simulink model "mrefrobotarm_modified_previous_y_previous_u_previous_ref"  (R2018b)
settings: Solver=FixedStepAuto  StartTime=0.0  StopTime=10  RelTol=1e-3  AbsTol=1e-6
undefined symbols (not defined in the file or in its folder): options, sfunxy2
libraries: neural x949, simulink x1
(part 25 of 31)

== system mrefrobotarm_modified_previous_y_previous_u_previous_ref/good_one/Layer 2/LW{2,1} ==
  "ad{2,1}" : Inport  PortDimensions=40
      mask Display: e = 0.06;c1 = [120 230 180]/255;c2 = ([120 230 180]+0)/(256+128);c3 = ([120 230 180]+128)/(256+128);patch([0 1 1 0],[0 0 1 1],c1);patch([0 1 1 1-e 1-e 0+e],[0 0 1 1-e 0+e 0+e],c2);patch([0 0 1 1-e 0+e 0+e],[0 1 1 1-e 1-e 0+e],c3);plot([0 1 1 0 0],[0 0 1 1 0]);
  "IW{2,1}(1,:)'" : Constant  Value=[-0.016177229018260623483183024973186547867953777313232421875;-0.096537565963239924116123802377842366695404052734375;-0.057321807043975082918141339405337930656969547271728515625;-0.33528888680619395312731967351282946765422821044921875;0.254536930512510084501087703756638802587985992431640625;0.160443440271881343495152805189718492329120635986328125;0.0298865770847444554847438524802782922051846981048583984375;-0.4905367415926971119688460021279752254486083984375;0.26949914824714371608394003487774170935153961181640625;0.279888712410184592460637986732763238251209259033203125;0.156475783700833093181614685818203724920749664306640625;0.427246473409241656060686409546178765594959259033203125;0.24892939455984686158984686699113808572292327880859375;0.2130922585627052778800560872696223668754100799560546875;0.09388320364746434443237177447372232563793659210205078125;-0.159198518445238190732737848520628176629543304443359375;0.01438968371043083081806113199263563728891313076019287109375;-0.0623226293562786637370010112135787494480609893798828125;0.403201394446350114275645637462730519473552703857421875;-1.209114934242264904895591826061718165874481201171875;0.8556447732028324981712330554728396236896514892578125;-0.124638437957925785060098178291809745132923126220703125;-0.87136147182802703436976798911928199231624603271484375;0.68733337340105526980238437317893840372562408447265625;0.08171188805447136827009302351143560372292995452880859375;0.62154317245998480512270134568098001182079315185546875;-0.142201082792390798292814224623725749552249908447265625;-0.058134677163346359929363416085834614932537078857421875;-0.0164424917618185388590301698741313884966075420379638671875;0.0377358747014499840144452491585980169475078582763671875;0.292289912994841805105039611589745618402957916259765625;0.76420559375889940412207579356618225574493408203125;-0.03434516763233952385547809171839617192745208740234375;-0.037602080927664947862520961052723578177392482757568359375;0.006550485557210122648796879474275556276552379131317138671875;0.04940602468184761286718043038490577600896358489990234375;-0.1541501906398750343374359772496973164379596710205078125;0.01187461167243125149950433439016705960966646671295166015625;0.01447827447317109363089659979095813469029963016510009765625;0.0172233274061301920576649848726447089575231075286865234375]
      mask Display: e = 0.06;c1 = [120 150 230]/255;c2 = ([120 150 230]+0)/383;c3 = ([120 150 230]+128)/383;patch([0 1 1 0],[0 0 1 1],c1);patch([0 1 1 1-e 1-e 0+e],[0 0 1 1-e 0+e 0+e],c2);patch([0 0 1 1-e 0+e 0+e],[0 1 1 1-e 1-e 0+e],c3);plot([0 1 1 0 0],[0 0 1 1 0]);disp('weights');
  Mux : Mux  Inputs=1
      mask Display: e = 0.06;c1 = [120 150 230]/255;c2 = ([120 150 230]+0)/383;c3 = ([120 150 230]+128)/383;patch([0 1 1 0],[0 0 1 1],c1);patch([0 1 1 1-e 1-e 0+e],[0 0 1 1-e 0+e 0+e],c2);patch([0 0 1 1-e 0+e 0+e],[0 1 1 1-e 1-e 0+e],c3);plot([0 1 1 0 0],[0 0 1 1 0]);disp('Mux');
  dotprod1 : neural/Weight Functions/dotprod
  "lz{2,1}" : Outport
      mask Display: e = 0.06;c1 = [120 230 180]/255;c2 = ([120 230 180]+0)/(256+128);c3 = ([120 230 180]+128)/(256+128);patch([0 1 1 0],[0 0 1 1],c1);patch([0 1 1 1-e 1-e 0+e],[0 0 1 1-e 0+e 0+e],c2);patch([0 0 1 1-e 0+e 0+e],[0 1 1 1-e 1-e 0+e],c3);plot([0 1 1 0 0],[0 0 1 1 0]);
  wires:
  "IW{2,1}(1,:)'"/1 -> dotprod1/1
  "ad{2,1}"/1 -> dotprod1/2
  dotprod1/1 -> Mux/1
  Mux/1 -> "lz{2,1}"/1

== system mrefrobotarm_modified_previous_y_previous_u_previous_ref/no_ss_error/Layer 1/Delays 1 ==
  "p{1}" : Inport  PortDimensions=10
      mask Display: e = 0.06;c1 = [120 230 180]/255;c2 = ([120 230 180]+0)/(256+128);c3 = ([120 230 180]+128)/(256+128);patch([0 1 1 0],[0 0 1 1],c1);patch([0 1 1 1-e 1-e 0+e],[0 0 1 1-e 0+e 0+e],c2);patch([0 0 1 1-e 0+e 0+e],[0 1 1 1-e 1-e 0+e],c3);plot([0 1 1 0 0],[0 0 1 1 0]);
  mux : Mux  Inputs=1
      mask Display: e = 0.06;c1 = [120 150 230]/255;c2 = ([120 150 230]+0)/383;c3 = ([120 150 230]+128)/383;patch([0 1 1 0],[0 0 1 1],c1);patch([0 1 1 1-e 1-e 0+e],[0 0 1 1-e 0+e 0+e],c2);patch([0 0 1 1-e 0+e 0+e],[0 1 1 1-e 1-e 0+e],c3);plot([0 1 1 0 0],[0 0 1 1 0]);disp('Mux')
  "pd{1,1}" : Outport
      mask Display: e = 0.06;c1 = [120 230 180]/255;c2 = ([120 230 180]+0)/(256+128);c3 = ([120 230 180]+128)/(256+128);patch([0 1 1 0],[0 0 1 1],c1);patch([0 1 1 1-e 1-e 0+e],[0 0 1 1-e 0+e 0+e],c2);patch([0 0 1 1-e 0+e 0+e],[0 1 1 1-e 1-e 0+e],c3);plot([0 1 1 0 0],[0 0 1 1 0]);
  wires:
  "p{1}"/1 -> mux/1
  mux/1 -> "pd{1,1}"/1

== system mrefrobotarm_modified_previous_y_previous_u_previous_ref/no_ss_error/Layer 1/IW{1,1} ==
  "pd{1,1}" : Inport  PortDimensions=10
      mask Display: e = 0.06;c1 = [120 230 180]/255;c2 = ([120 230 180]+0)/(256+128);c3 = ([120 230 180]+128)/(256+128);patch([0 1 1 0],[0 0 1 1],c1);patch([0 1 1 1-e 1-e 0+e],[0 0 1 1-e 0+e 0+e],c2);patch([0 0 1 1-e 0+e 0+e],[0 1 1 1-e 1-e 0+e],c3);plot([0 1 1 0 0],[0 0 1 1 0]);
  "IW{1,1}(1,:)'" : Constant  Value=[0.52268284589696356601251636675442568957805633544921875;0.26452162295619441323424325673840939998626708984375;0.6302383946003129455704083738964982330799102783203125;0.1670856108177140864068377368312212638556957244873046875;1.6390040056115242617096328103798441588878631591796875;-0.8986878651207874657558249964495189487934112548828125;-1.114512508252162081845426655490882694721221923828125;-0.423456516896269619110171333886682987213134765625;0.20198751257098113143229056731797754764556884765625;0.47139361413845304316083684170735068619251251220703125]
      mask Display: e = 0.06;c1 = [120 150 230]/255;c2 = ([120 150 230]+0)/383;c3 = ([120 150 230]+128)/383;patch([0 1 1 0],[0 0 1 1],c1);patch([0 1 1 1-e 1-e 0+e],[0 0 1 1-e 0+e 0+e],c2);patch([0 0 1 1-e 0+e 0+e],[0 1 1 1-e 1-e 0+e],c3);plot([0 1 1 0 0],[0 0 1 1 0]);disp('Weights');
  "IW{1,1}(10,:)'" : Constant  Value=[1.2597231626400127169063125620596110820770263671875;0.331393970410923388580926030044793151319026947021484375;-0.052791829980691880319643161101339501328766345977783203125;0.3149576319875482255383758456446230411529541015625;0.55511068393909435148003694848739542067050933837890625;0.96721718074699747358380363948526792228221893310546875;0.9771018529696899879155580492806620895862579345703125;-0.269806974086425788161847094670520164072513580322265625;1.5151280312247499271194328684941865503787994384765625;-0.1203640526482755712667227498968713916838169097900390625]
      mask Display: e = 0.06;c1 = [120 150 230]/255;c2 = ([120 150 230]+0)/383;c3 = ([120 150 230]+128)/383;patch([0 1 1 0],[0 0 1 1],c1);patch([0 1 1 1-e 1-e 0+e],[0 0 1 1-e 0+e 0+e],c2);patch([0 0 1 1-e 0+e 0+e],[0 1 1 1-e 1-e 0+e],c3);plot([0 1 1 0 0],[0 0 1 1 0]);disp('Weights');
  "IW{1,1}(11,:)'" : Constant  Value=[-1.0743295819324780726589096957468427717685699462890625;1.1501577563757912070485645017470233142375946044921875;-0.86958362725818016958356793111306615173816680908203125;0.29387617229097073856536326275090686976909637451171875;1.8821297501686731212799941204139031469821929931640625;-0.8969617337271689194722057436592876911163330078125;-0.153795010052089897722993327988660894334316253662109375;-0.424733827549765796671721318489289842545986175537109375;1.58320681511508354333273018710315227508544921875;0.1647340537904307955496818749452359043061733245849609375]
      mask Display: e = 0.06;c1 = [120 150 230]/255;c2 = ([120 150 230]+0)/383;c3 = ([120 150 230]+128)/383;patch([0 1 1 0],[0 0 1 1],c1);patch([0 1 1 1-e 1-e 0+e],[0 0 1 1-e 0+e 0+e],c2);patch([0 0 1 1-e 0+e 0+e],[0 1 1 1-e 1-e 0+e],c3);plot([0 1 1 0 0],[0 0 1 1 0]);disp('Weights');
  "IW{1,1}(12,:)'" : Constant  Value=[-0.180456952373312662363247227403917349874973297119140625;-0.9119322220681633783812003457569517195224761962890625;-0.7206769917408870629316197664593346416950225830078125;0.51991005391813416292023930509458296000957489013671875;1.3325131012939082086887765399296768009662628173828125;1.2068826405339387886073154732002876698970794677734375;-0.25797017784359310699215939166606403887271881103515625;-0.5702990169558226352108931678230874240398406982421875;-1.0030700930944382864851149861351586878299713134765625;-0.8022722469174292658777858378016389906406402587890625]
      mask Display: e = 0.06;c1 = [120 150 230]/255;c2 = ([120 150 230]+0)/383;c3 = ([120 150 230]+128)/383;patch([0 1 1 0],[0 0 1 1],c1);patch([0 1 1 1-e 1-e 0+e],[0 0 1 1-e 0+e 0+e],c2);patch([0 0 1 1-e 0+e 0+e],[0 1 1 1-e 1-e 0+e],c3);plot([0 1 1 0 0],[0 0 1 1 0]);disp('Weights');
  "IW{1,1}(13,:)'" : Constant  Value=[1.587500865720722575957779554300941526889801025390625;-0.4136221707058511665167088722228072583675384521484375;-0.52639486621294195867193366211722604930400848388671875;0.6173652998952949833011416558292694389820098876953125;0.3804309528306466514635530984378419816493988037109375;0.43292517299477883963021440649754367768764495849609375;-0.059184167845455604162197005280177108943462371826171875;-0.520069104891264455403643296449445188045501708984375;-0.262239897051457171439636795184924267232418060302734375;0.04362502873940894698723269584661466069519519805908203125]
      mask Display: e = 0.06;c1 = [120 150 230]/255;c2 = ([120 150 230]+0)/383;c3 = ([120 150 230]+128)/383;patch([0 1 1 0],[0 0 1 1],c1);patch([0 1 1 1-e 1-e 0+e],[0 0 1 1-e 0+e 0+e],c2);patch([0 0 1 1-e 0+e 0+e],[0 1 1 1-e 1-e 0+e],c3);plot([0 1 1 0 0],[0 0 1 1 0]);disp('Weights');
  "IW{1,1}(14,:)'" : Constant  Value=[0.15678260333455951158754260177374817430973052978515625;-0.2830214288855901205721465885289944708347320556640625;-0.57337904103334758065813048233394511044025421142578125;-0.58607875125629771417834490421228110790252685546875;0.9772944325289447675686460570432245731353759765625;-1.0061880783424668184267147807986475527286529541015625;0.12184461872279016281250818565240479074418544769287109375;-0.093833824658861642031837391186854802072048187255859375;0.5364472996047109365491678545367904007434844970703125;0.324149798798010035927319449911010451614856719970703125]
      mask Display: e = 0.06;c1 = [120 150 230]/255;c2 = ([120 150 230]+0)/383;c3 = ([120 150 230]+128)/383;patch([0 1 1 0],[0 0 1 1],c1);patch([0 1 1 1-e 1-e 0+e],[0 0 1 1-e 0+e 0+e],c2);patch([0 0 1 1-e 0+e 0+e],[0 1 1 1-e 1-e 0+e],c3);plot([0 1 1 0 0],[0 0 1 1 0]);disp('Weights');
  "IW{1,1}(15,:)'" : Constant  Value=[-0.597168529912007528537287726067006587982177734375;-0.26877976344490683846544243351672776043415069580078125;-0.4210029627419034081725612850277684628963470458984375;-0.895478281549339616418592413538135588169097900390625;-0.185230952547398686203194984045694582164287567138671875;-0.202950183795940486408682090768706984817981719970703125;0.57595042618450376092908982172957621514797210693359375;-0.63455501901511734974548062382382340729236602783203125;-0.979057802580790781377118037198670208454132080078125;-0.886842867770659015747014564112760126590728759765625]
      mask Display: e = 0.06;c1 = [120 150 230]/255;c2 = ([120 150 230]+0)/383;c3 = ([120 150 230]+128)/383;patch([0 1 1 0],[0 0 1 1],c1);patch([0 1 1 1-e 1-e 0+e],[0 0 1 1-e 0+e 0+e],c2);patch([0 0 1 1-e 0+e 0+e],[0 1 1 1-e 1-e 0+e],c3);plot([0 1 1 0 0],[0 0 1 1 0]);disp('Weights');
  "IW{1,1}(16,:)'" : Constant  Value=[-1.4434083519231160064322239122702740132808685302734375;-0.89746723355772584085343623883090913295745849609375;0.468903432219882787546083591223577968776226043701171875;0.5235125480188809188319964960101060569286346435546875;1.030194455855783619568910580710507929325103759765625;0.2410749054790011225435364394797943532466888427734375;-0.020026318196021346274005026089071179740130901336669921875;0.12832652380476472497861095689586363732814788818359375;0.1470700867800898148374244556180201470851898193359375;0.9743179738880478613083369054947979748249053955078125]
      mask Display: e = 0.06;c1 = [120 150 230]/255;c2 = ([120 150 230]+0)/383;c3 = ([120 150 230]+128)/383;patch([0 1 1 0],[0 0 1 1],c1);patch([0 1 1 1-e 1-e 0+e],[0 0 1 1-e 0+e 0+e],c2);patch([0 0 1 1-e 0+e 0+e],[0 1 1 1-e 1-e 0+e],c3);plot([0 1 1 0 0],[0 0 1 1 0]);disp('Weights');
  "IW{1,1}(17,:)'" : Constant  Value=[-1.998604254806128910360030204174108803272247314453125;0.781327841746925155774761151405982673168182373046875;1.104473632181291353759888806962408125400543212890625;0.6244245059941342379516981964115984737873077392578125;-1.8270110679777420426006528941798023879528045654296875;1.57781831173188979988708524615503847599029541015625;0.17040001620197653409150007064454257488250732421875;0.343192753239213887983538597836741246283054351806640625;0.3575702811109369161357562916236929595470428466796875;-0.040126214462137231586691399343180819414556026458740234375]
      mask Display: e = 0.06;c1 = [120 150 230]/255;c2 = ([120 150 230]+0)/383;c3 = ([120 150 230]+128)/383;patch([0 1 1 0],[0 0 1 1],c1);patch([0 1 1 1-e 1-e 0+e],[0 0 1 1-e 0+e 0+e],c2);patch([0 0 1 1-e 0+e 0+e],[0 1 1 1-e 1-e 0+e],c3);plot([0 1 1 0 0],[0 0 1 1 0]);disp('Weights');
  "IW{1,1}(18,:)'" : Constant  Value=[0.86997594199966099548504416816285811364650726318359375;-0.892679254067974436992471964913420379161834716796875;-0.04449260537774453461157264655412291176617145538330078125;0.9604625897041871862569450968294404447078704833984375;-0.30233191807039239140664221849874593317508697509765625;-1.8516467076794871360334582277573645114898681640625;1.262375674633811950542394697549752891063690185546875;0.28182724484288634858586419795756228268146514892578125;-0.58009991273124372757052924498566426336765289306640625;0.23561111386226318842318505630828440189361572265625]
      mask Display: e = 0.06;c1 = [120 150 230]/255;c2 = ([120 150 230]+0)/383;c3 = ([120 150 230]+128)/383;patch([0 1 1 0],[0 0 1 1],c1);patch([0 1 1 1-e 1-e 0+e],[0 0 1 1-e 0+e 0+e],c2);patch([0 0 1 1-e 0+e 0+e],[0 1 1 1-e 1-e 0+e],c3);plot([0 1 1 0 0],[0 0 1 1 0]);disp('Weights');
  "IW{1,1}(19,:)'" : Constant  Value=[-0.32234142998081638520346814402728341519832611083984375;-0.17724685528195960326769409221014939248561859130859375;0.91705950576351480396652959825587458908557891845703125;0.51157014029427372303615584314684383571147918701171875;0.1887748557125419057722837123947101645171642303466796875;-0.2402553739407127519900342349501443095505237579345703125;-1.022254798633368100269080969155766069889068603515625;0.96340859299408798666064512872253544628620147705078125;-0.49104755155709056690938041356275789439678192138671875;0.478083620793313401886592828304856084287166595458984375]
      mask Display: e = 0.06;c1 = [120 150 230]/255;c2 = ([120 150 230]+0)/383;c3 = ([120 150 230]+128)/383;patch([0 1 1 0],[0 0 1 1],c1);patch([0 1 1 1-e 1-e 0+e],[0 0 1 1-e 0+e 0+e],c2);patch([0 0 1 1-e 0+e 0+e],[0 1 1 1-e 1-e 0+e],c3);plot([0 1 1 0 0],[0 0 1 1 0]);disp('Weights');
  "IW{1,1}(2,:)'" : Constant  Value=[1.1125574577235786133400097241974435746669769287109375;-1.035051422440350421538823866285383701324462890625;0.83885387255288323959945273600169457495212554931640625;0.0953643030795100210550430119837983511388301849365234375;-1.781602566605932747023643969441764056682586669921875;1.494386247798205058501253006397746503353118896484375;-0.4333392812288605622228487845859490334987640380859375;0.0661252406685951255038702356614521704614162445068359375;-1.1169056384897666500677360090776346623897552490234375;-0.049751712353421302659217673181046848185360431671142578125]
      mask Display: e = 0.06;c1 = [120 150 230]/255;c2 = ([120 150 230]+0)/383;c3 = ([120 150 230]+128)/383;patch([0 1 1 0],[0 0 1 1],c1);patch([0 1 1 1-e 1-e 0+e],[0 0 1 1-e 0+e 0+e],c2);patch([0 0 1 1-e 0+e 0+e],[0 1 1 1-e 1-e 0+e],c3);plot([0 1 1 0 0],[0 0 1 1 0]);disp('Weights');
  "IW{1,1}(20,:)'" : Constant  Value=[-1.0550509035035673388591703769634477794170379638671875;1.47722490339520096114256375585682690143585205078125;0.3866391515635438924647360181552357971668243408203125;1.0983933950853543848324989085085690021514892578125;-0.2221131732843392991849640338841709308326244354248046875;0.86580731540057176420788209725287742912769317626953125;-0.298216110609449358559430720561067573726177215576171875;0.25209568597034770487397281613084487617015838623046875;0.589275825413892118120884333620779216289520263671875;0.34374689982705775026516903380979783833026885986328125]
      mask Display: e = 0.06;c1 = [120 150 230]/255;c2 = ([120 150 230]+0)/383;c3 = ([120 150 230]+128)/383;patch([0 1 1 0],[0 0 1 1],c1);patch([0 1 1 1-e 1-e 0+e],[0 0 1 1-e 0+e 0+e],c2);patch([0 0 1 1-e 0+e 0+e],[0 1 1 1-e 1-e 0+e],c3);plot([0 1 1 0 0],[0 0 1 1 0]);disp('Weights');
  "IW{1,1}(3,:)'" : Constant  Value=[-0.1998919188007486635871856606172514148056507110595703125;-1.0956278610275147489261371447355486452579498291015625;-1.630336875325356427168799200444482266902923583984375;-1.099723709930339854423664291971363127231597900390625;1.96708475838372809363363558077253401279449462890625;-0.7724713323078635784924017571029253304004669189453125;2.273417873343792194873458356596529483795166015625;1.1251114038756855340039919610717333853244781494140625;1.2772586657711808566517674989881925284862518310546875;0.19164022257996748965780398066272027790546417236328125]
      mask Display: e = 0.06;c1 = [120 150 230]/255;c2 = ([120 150 230]+0)/383;c3 = ([120 150 230]+128)/383;patch([0 1 1 0],[0 0 1 1],c1);patch([0 1 1 1-e 1-e 0+e],[0 0 1 1-e 0+e 0+e],c2);patch([0 0 1 1-e 0+e 0+e],[0 1 1 1-e 1-e 0+e],c3);plot([0 1 1 0 0],[0 0 1 1 0]);disp('Weights');
  "IW{1,1}(4,:)'" : Constant  Value=[-1.2772127548669460761487925992696546018123626708984375;-0.414613370828340099816244901376194320619106292724609375;1.40626694606605884274586060200817883014678955078125;0.11057759758240502667714366680229431949555873870849609375;1.6069989829620607846294433329603634774684906005859375;-0.478564693118000150651170088167418725788593292236328125;0.09863218609341216358554760290644480846822261810302734375;-0.2081346556125294455785734726305236108601093292236328125;-0.6534127800186768642021206687786616384983062744140625;-0.867836103660213353805374936200678348541259765625]
      mask Display: e = 0.06;c1 = [120 150 230]/255;c2 = ([120 150 230]+0)/383;c3 = ([120 150 230]+128)/383;patch([0 1 1 0],[0 0 1 1],c1);patch([0 1 1 1-e 1-e 0+e],[0 0 1 1-e 0+e 0+e],c2);patch([0 0 1 1-e 0+e 0+e],[0 1 1 1-e 1-e 0+e],c3);plot([0 1 1 0 0],[0 0 1 1 0]);disp('Weights');
  "IW{1,1}(5,:)'" : Constant  Value=[-0.67657225807134546702314992216997779905796051025390625;-0.2346639369608422842627959425954031758010387420654296875;0.44159934201549677634801582826185040175914764404296875;0.9069623237870125809223509349976666271686553955078125;-0.29434057215699038767553474826854653656482696533203125;-0.65745407442928505137302863658987917006015777587890625;0.24355260585492810587737722016754560172557830810546875;-0.309437933100902562433276443698559887707233428955078125;-0.27819664327048077012705107335932552814483642578125;1.659439867511534050237287374329753220081329345703125]
      mask Display: e = 0.06;c1 = [120 150 230]/255;c2 = ([120 150 230]+0)/383;c3 = ([120 150 230]+128)/383;patch([0 1 1 0],[0 0 1 1],c1);patch([0 1 1 1-e 1-e 0+e],[0 0 1 1-e 0+e 0+e],c2);patch([0 0 1 1-e 0+e 0+e],[0 1 1 1-e 1-e 0+e],c3);plot([0 1 1 0 0],[0 0 1 1 0]);disp('Weights');
  "IW{1,1}(6,:)'" : Constant  Value=[-0.63274484531872510206795823251013644039630889892578125;-1.09588525241094369988559265038929879665374755859375;0.463661599302709059866600682653370313346385955810546875;-0.466312531851492406698156401034793816506862640380859375;0.1854504718639355953513359054340980947017669677734375;1.497685414012905891212312781135551631450653076171875;0.281762713901031858210188829616527073085308074951171875;0.59707615716941131456252378484350629150867462158203125;-1.578556705452232034048165587591938674449920654296875;-0.91641682544859881520693534184829331934452056884765625]
      mask Display: e = 0.06;c1 = [120 150 230]/255;c2 = ([120 150 230]+0)/383;c3 = ([120 150 230]+128)/383;patch([0 1 1 0],[0 0 1 1],c1);patch([0 1 1 1-e 1-e 0+e],[0 0 1 1-e 0+e 0+e],c2);patch([0 0 1 1-e 0+e 0+e],[0 1 1 1-e 1-e 0+e],c3);plot([0 1 1 0 0],[0 0 1 1 0]);disp('Weights');
  "IW{1,1}(7,:)'" : Constant  Value=[0.4124484193097590623011683419463224709033966064453125;1.6123019995529490611119172172038815915584564208984375;0.854771910029324288871066528372466564178466796875;2.038794023702274582632298915996216237545013427734375;-0.51977571159315993920557730234577320516109466552734375;-2.48024327230679642042332488927058875560760498046875;-1.5524874401718165017882711254060268402099609375;-0.5499061093922141818524096379405818879604339599609375;0.7764604915715833666212120078853331506252288818359375;-0.477045060227799189167541271672234870493412017822265625]
      mask Display: e = 0.06;c1 = [120 150 230]/255;c2 = ([120 150 230]+0)/383;c3 = ([120 150 230]+128)/383;patch([0 1 1 0],[0 0 1 1],c1);patch([0 1 1 1-e 1-e 0+e],[0 0 1 1-e 0+e 0+e],c2);patch([0 0 1 1-e 0+e 0+e],[0 1 1 1-e 1-e 0+e],c3);plot([0 1 1 0 0],[0 0 1 1 0]);disp('Weights');
  "IW{1,1}(8,:)'" : Constant  Value=[0.207085959866739444112937462705303914844989776611328125;1.0829233288839079651921792901703156530857086181640625;-0.139610716808303003677593778775190003216266632080078125;-0.43072901796916607253251640941016376018524169921875;-0.2733103643586412001553753725602291524410247802734375;-0.4479654798819308059165678059798665344715118408203125;-0.292329437772251010674295912394882179796695709228515625;0.1397490932171858990518131804492441006004810333251953125;0.369801551336038369921510593485436402261257171630859375;-0.48701713915047106784328434514463879168033599853515625]
      mask Display: e = 0.06;c1 = [120 150 230]/255;c2 = ([120 150 230]+0)/383;c3 = ([120 150 230]+128)/383;patch([0 1 1 0],[0 0 1 1],c1);patch([0 1 1 1-e 1-e 0+e],[0 0 1 1-e 0+e 0+e],c2);patch([0 0 1 1-e 0+e 0+e],[0 1 1 1-e 1-e 0+e],c3);plot([0 1 1 0 0],[0 0 1 1 0]);disp('Weights');
  "IW{1,1}(9,:)'" : Constant  Value=[-0.276800130397536314763584641696070320904254913330078125;0.9085992318130615696958329863264225423336029052734375;0.97038321195353904879965512009221129119396209716796875;-0.449245786675241565166771806616452522575855255126953125;-0.001382483860408670849062584551347754313610494136810302734375;0.1422487805634587709757710172198130749166011810302734375;0.55617839542495506321984066744334995746612548828125;0.23460571971346777520039950104546733200550079345703125;0.87316002745057141876117157153203152120113372802734375;0.3721153994530281838848395636887289583683013916015625]
      mask Display: e = 0.06;c1 = [120 150 230]/255;c2 = ([120 150 230]+0)/383;c3 = ([120 150 230]+128)/383;patch([0 1 1 0],[0 0 1 1],c1);patch([0 1 1 1-e 1-e 0+e],[0 0 1 1-e 0+e 0+e],c2);patch([0 0 1 1-e 0+e 0+e],[0 1 1 1-e 1-e 0+e],c3);plot([0 1 1 0 0],[0 0 1 1 0]);disp('Weights');
  Mux : Mux  Inputs=20
      mask Display: e = 0.06;c1 = [120 150 230]/255;c2 = ([120 150 230]+0)/383;c3 = ([120 150 230]+128)/383;patch([0 1 1 0],[0 0 1 1],c1);patch([0 1 1 1-e 1-e 0+e],[0 0 1 1-e 0+e 0+e],c2);patch([0 0 1 1-e 0+e 0+e],[0 1 1 1-e 1-e 0+e],c3);plot([0 1 1 0 0],[0 0 1 1 0]);disp('Mux');
  dotprod{1..20} (20 alike) : neural/Weight Functions/dotprod
  "iz{1,1}" : Outport
      mask Display: e = 0.06;c1 = [120 230 180]/255;c2 = ([120 230 180]+0)/(256+128);c3 = ([120 230 180]+128)/(256+128);patch([0 1 1 0],[0 0 1 1],c1);patch([0 1 1 1-e 1-e 0+e],[0 0 1 1-e 0+e 0+e],c2);patch([0 0 1 1-e 0+e 0+e],[0 1 1 1-e 1-e 0+e],c3);plot([0 1 1 0 0],[0 0 1 1 0]);
  wires:
  "IW{1,1}(1,:)'"/1 -> dotprod1/1
  "pd{1,1}"/1 -> dotprod1/2, dotprod2/2, dotprod3/2, dotprod4/2, dotprod5/2, dotprod6/2, dotprod7/2, dotprod8/2, dotprod9/2, dotprod10/2, dotprod11/2, dotprod12/2, dotprod13/2, dotprod14/2, dotprod15/2, dotprod16/2, dotprod17/2, dotprod18/2, dotprod19/2, dotprod20/2
  dotprod1/1 -> Mux/1
  "IW{1,1}(2,:)'"/1 -> dotprod2/1
  dotprod2/1 -> Mux/2
  "IW{1,1}(3,:)'"/1 -> dotprod3/1
  dotprod3/1 -> Mux/3
  "IW{1,1}(4,:)'"/1 -> dotprod4/1
  dotprod4/1 -> Mux/4
  "IW{1,1}(5,:)'"/1 -> dotprod5/1
  dotprod5/1 -> Mux/5
  "IW{1,1}(6,:)'"/1 -> dotprod6/1
  dotprod6/1 -> Mux/6
  "IW{1,1}(7,:)'"/1 -> dotprod7/1
  dotprod7/1 -> Mux/7
  "IW{1,1}(8,:)'"/1 -> dotprod8/1
  dotprod8/1 -> Mux/8
  "IW{1,1}(9,:)'"/1 -> dotprod9/1
  dotprod9/1 -> Mux/9
  "IW{1,1}(10,:)'"/1 -> dotprod10/1
  dotprod10/1 -> Mux/10
  "IW{1,1}(11,:)'"/1 -> dotprod11/1
  dotprod11/1 -> Mux/11
  "IW{1,1}(12,:)'"/1 -> dotprod12/1
  dotprod12/1 -> Mux/12
  "IW{1,1}(13,:)'"/1 -> dotprod13/1
  dotprod13/1 -> Mux/13
  "IW{1,1}(14,:)'"/1 -> dotprod14/1
  dotprod14/1 -> Mux/14
  "IW{1,1}(15,:)'"/1 -> dotprod15/1
  dotprod15/1 -> Mux/15
  "IW{1,1}(16,:)'"/1 -> dotprod16/1
  dotprod16/1 -> Mux/16
  "IW{1,1}(17,:)'"/1 -> dotprod17/1
  dotprod17/1 -> Mux/17
  "IW{1,1}(18,:)'"/1 -> dotprod18/1
  dotprod18/1 -> Mux/18
  "IW{1,1}(19,:)'"/1 -> dotprod19/1
  dotprod19/1 -> Mux/19
  "IW{1,1}(20,:)'"/1 -> dotprod20/1
  dotprod20/1 -> Mux/20
  Mux/1 -> "iz{1,1}"/1

== system mrefrobotarm_modified_previous_y_previous_u_previous_ref/no_ss_error/Layer 2/Delays 1 ==
  "p{2}" : Inport  PortDimensions=20
      mask Display: e = 0.06;c1 = [120 230 180]/255;c2 = ([120 230 180]+0)/(256+128);c3 = ([120 230 180]+128)/(256+128);patch([0 1 1 0],[0 0 1 1],c1);patch([0 1 1 1-e 1-e 0+e],[0 0 1 1-e 0+e 0+e],c2);patch([0 0 1 1-e 0+e 0+e],[0 1 1 1-e 1-e 0+e],c3);plot([0 1 1 0 0],[0 0 1 1 0]);
  mux : Mux  Inputs=1
      mask Display: e = 0.06;c1 = [120 150 230]/255;c2 = ([120 150 230]+0)/383;c3 = ([120 150 230]+128)/383;patch([0 1 1 0],[0 0 1 1],c1);patch([0 1 1 1-e 1-e 0+e],[0 0 1 1-e 0+e 0+e],c2);patch([0 0 1 1-e 0+e 0+e],[0 1 1 1-e 1-e 0+e],c3);plot([0 1 1 0 0],[0 0 1 1 0]);disp('Mux')
  "pd{2,1}" : Outport
      mask Display: e = 0.06;c1 = [120 230 180]/255;c2 = ([120 230 180]+0)/(256+128);c3 = ([120 230 180]+128)/(256+128);patch([0 1 1 0],[0 0 1 1],c1);patch([0 1 1 1-e 1-e 0+e],[0 0 1 1-e 0+e 0+e],c2);patch([0 0 1 1-e 0+e 0+e],[0 1 1 1-e 1-e 0+e],c3);plot([0 1 1 0 0],[0 0 1 1 0]);
  wires:
  "p{2}"/1 -> mux/1
  mux/1 -> "pd{2,1}"/1

== system mrefrobotarm_modified_previous_y_previous_u_previous_ref/no_ss_error/Layer 2/LW{2,1} ==
  "ad{2,1}" : Inport  PortDimensions=20
      mask Display: e = 0.06;c1 = [120 230 180]/255;c2 = ([120 230 180]+0)/(256+128);c3 = ([120 230 180]+128)/(256+128);patch([0 1 1 0],[0 0 1 1],c1);patch([0 1 1 1-e 1-e 0+e],[0 0 1 1-e 0+e 0+e],c2);patch([0 0 1 1-e 0+e 0+e],[0 1 1 1-e 1-e 0+e],c3);plot([0 1 1 0 0],[0 0 1 1 0]);
  "IW{2,1}(1,:)'" : Constant  Value=[0.6246526241400747192500375604140572249889373779296875;0.038795776017597809193215852019420708529651165008544921875;0.40820713704172051361496187382726930081844329833984375;-1.4171707757667435512161091537564061582088470458984375;-0.415391421107700720138922179103246890008449554443359375;0.097006870602628192390426420388394035398960113525390625;1.070731206069215346587952808476984500885009765625;-0.52730678401085506745715747456415556371212005615234375;0.244126131180451955149379728027270175516605377197265625;-0.41916710117515665334764207727857865393161773681640625;0.34311023554087494158437721125665120780467987060546875;1.836752047915414021161950586247257888317108154296875;0.1934653332798478009291187618146068416535854339599609375;-0.35462545465756367679688310090568847954273223876953125;0.3045310972162822427122819135547615587711334228515625;0.01699944495094095342491158362463465891778469085693359375;0.8313837407592321593341466723359189927577972412109375;-0.2664706811988641899091589948511682450771331787109375;-0.48454175102535634866995906122610904276371002197265625;0.039137110510804450080879490769802941940724849700927734375]
      mask Display: e = 0.06;c1 = [120 150 230]/255;c2 = ([120 150 230]+0)/383;c3 = ([120 150 230]+128)/383;patch([0 1 1 0],[0 0 1 1],c1);patch([0 1 1 1-e 1-e 0+e],[0 0 1 1-e 0+e 0+e],c2);patch([0 0 1 1-e 0+e 0+e],[0 1 1 1-e 1-e 0+e],c3);plot([0 1 1 0 0],[0 0 1 1 0]);disp('weights');
  "IW{2,1}(10,:)'" : Constant  Value=[0.43336819186250219448908183039748109877109527587890625;-0.982821758980740423083943824167363345623016357421875;0.841923599707687486670693033374845981597900390625;-0.50959030652609971223654383720713667571544647216796875;-0.542439947616161877164131510653533041477203369140625;0.339280306809299159187531813586247153580188751220703125;0.70641710426591874938395676508662290871143341064453125;0.26157463775194944588520229444839060306549072265625;0.15039361498558478924536530030309222638607025146484375;0.2307066340758537614785694813690497539937496185302734375;-0.877705170560429959181192316464148461818695068359375;-0.1978171214243842346292012734920717775821685791015625;-0.64840760673419606252565472459536977112293243408203125;-0.4302029122337589495117526894318871200084686279296875;0.22056179001425169072803100789315067231655120849609375;0.0527296119499969517807613783588749356567859649658203125;-0.2618395551117462805024160843458957970142364501953125;0.218769394556477980717801301580038852989673614501953125;-0.466834901204433549981587248112191446125507354736328125;0.98285365981584937866699647202040068805217742919921875]
      mask Display: e = 0.06;c1 = [120 150 230]/255;c2 = ([120 150 230]+0)/383;c3 = ([120 150 230]+128)/383;patch([0 1 1 0],[0 0 1 1],c1);patch([0 1 1 1-e 1-e 0+e],[0 0 1 1-e 0+e 0+e],c2);patch([0 0 1 1-e 0+e 0+e],[0 1 1 1-e 1-e 0+e],c3);plot([0 1 1 0 0],[0 0 1 1 0]);disp('weights');
  "IW{2,1}(2,:)'" : Constant  Value=[-0.76551284609604641762103938162908889353275299072265625;0.129145585277098629006786723039112985134124755859375;0.44767402081057749985149030180764384567737579345703125;1.0050317178177461396870739918085746467113494873046875;0.493924502049837566008960720864706672728061676025390625;-1.2811917787235789223387882884708233177661895751953125;-0.0044713580952384958389078661866733455099165439605712890625;-0.92153573554992396221763328867382369935512542724609375;-0.020634218795010837721459751037400565110146999359130859375;0.195947930299892714156584361262503080070018768310546875;-0.57929769073577908056194019081885926425457000732421875;-0.6745480567676140903898840406327508389949798583984375;-0.37201989589266581948123757683788426220417022705078125;-0.04511008335553857995225968124941573478281497955322265625;0.0504365160942186474546389263196033425629138946533203125;-1.063776506503057550645507944864220917224884033203125;-0.45769552699465443357240701516275294125080108642578125;-1.2113433040788532668585730789345689117908477783203125;-0.11827178691914362607118249570703483186662197113037109375;-0.236030646388771525590044575437786988914012908935546875]
      mask Display: e = 0.06;c1 = [120 150 230]/255;c2 = ([120 150 230]+0)/383;c3 = ([120 150 230]+128)/383;patch([0 1 1 0],[0 0 1 1],c1);patch([0 1 1 1-e 1-e 0+e],[0 0 1 1-e 0+e 0+e],c2);patch([0 0 1 1-e 0+e 0+e],[0 1 1 1-e 1-e 0+e],c3);plot([0 1 1 0 0],[0 0 1 1 0]);disp('weights');
  "IW{2,1}(3,:)'" : Constant  Value=[-0.314067791204970803153884162384201772511005401611328125;0.313284166018203802384078926479560323059558868408203125;-1.112516761141086885089634961332194507122039794921875;-0.436508420587207679464114562506438232958316802978515625;-0.825760450935524747961835601017810404300689697265625;0.01340720143956012667951771533125793212093412876129150390625;-0.41239637577193211104287229318288154900074005126953125;0.25923803926188870860869428724981844425201416015625;0.55080492699819372237612924436689354479312896728515625;0.66050018331517013070453003820148296654224395751953125;0.18586477009082169598030986890080384910106658935546875;-0.11975989301560673039315219057243666611611843109130859375;-0.64920263482511553210230204058461822569370269775390625;-0.0084725366529001290560874082302689203061163425445556640625;0.436306856808362564237313563353382050991058349609375;-0.436750875850537900735304219779209233820438385009765625;-1.6732536600374425805881628548377193510532379150390625;0.074227476317377416581422266972367651760578155517578125;-0.156740773602614458237525241202092729508876800537109375;-0.160849982695082160955024619397590868175029754638671875]
      mask Display: e = 0.06;c1 = [120 150 230]/255;c2 = ([120 150 230]+0)/383;c3 = ([120 150 230]+128)/383;patch([0 1 1 0],[0 0 1 1],c1);patch([0 1 1 1-e 1-e 0+e],[0 0 1 1-e 0+e 0+e],c2);patch([0 0 1 1-e 0+e 0+e],[0 1 1 1-e 1-e 0+e],c3);plot([0 1 1 0 0],[0 0 1 1 0]);disp('weights');
  "IW{2,1}(4,:)'" : Constant  Value=[-0.1953818262767609004182389753623283468186855316162109375;0.1672530029882540458796569282640120945870876312255859375;-0.1676354655624912037836793388123624026775360107421875;0.56691397826103917534368292763247154653072357177734375;0.76013009223308924955375687204650603234767913818359375;0.64763762026116200587466664728708565235137939453125;0.12142554979095616929374301662392099387943744659423828125;-0.1408209411656707599203031122669926844537258148193359375;-0.1406444916578379611404869820034946314990520477294921875;-0.73643827671563866221760008556884713470935821533203125;0.452911361158982617158841321725049056112766265869140625;0.72592962236882885296296308297314681112766265869140625;0.67806005667402724501613420216017402708530426025390625;-0.2418495788419389447287954908460960723459720611572265625;0.488803601136513776737047010101377964019775390625;0.09816642903615267756745055294231860898435115814208984375;-0.9601818968046871294319544176687486469745635986328125;-0.051387867235737648419213741135536110959947109222412109375;0.278947277527112902362205204553902149200439453125;-0.53441342110937462006603482222999446094036102294921875]
      mask Display: e = 0.06;c1 = [120 150 230]/255;c2 = ([120 150 230]+0)/383;c3 = ([120 150 230]+128)/383;patch([0 1 1 0],[0 0 1 1],c1);patch([0 1 1 1-e 1-e 0+e],[0 0 1 1-e 0+e 0+e],c2);patch([0 0 1 1-e 0+e 0+e],[0 1 1 1-e 1-e 0+e],c3);plot([0 1 1 0 0],[0 0 1 1 0]);disp('weights');
  "IW{2,1}(5,:)'" : Constant  Value=[-0.80402480350838623213149958246503956615924835205078125;0.9994673608273767495546735517564229667186737060546875;-0.66014139768686497244942756879027001559734344482421875;-1.34949057026407093218267618794925510883331298828125;-0.322417017208455891630336509479093365371227264404296875;0.1310637229823681249030187245807610452175140380859375;-0.50259326990763764086977971601299941539764404296875;-0.83804248562761907148654927368625067174434661865234375;0.3332765829657347023129432272980920970439910888671875;-0.0566777687495015058960490250683506019413471221923828125;0.037446976489596543735682843134782160632312297821044921875;0.6975490190955910829728736644028685986995697021484375;0.038757921922094283606607945102950907312333583831787109375;0.08227323375619004230951958334117080084979534149169921875;0.3428176055717973014225208316929638385772705078125;0.286962719331971094494093676985357888042926788330078125;-1.30079300128597452612666529603302478790283203125;0.351280862578072172741627809955389238893985748291015625;0.385744573352316655334703909829840995371341705322265625;0.84394839256656439818726767043699510395526885986328125]
      mask Display: e = 0.06;c1 = [120 150 230]/255;c2 = ([120 150 230]+0)/383;c3 = ([120 150 230]+128)/383;patch([0 1 1 0],[0 0 1 1],c1);patch([0 1 1 1-e 1-e 0+e],[0 0 1 1-e 0+e 0+e],c2);patch([0 0 1 1-e 0+e 0+e],[0 1 1 1-e 1-e 0+e],c3);plot([0 1 1 0 0],[0 0 1 1 0]);disp('weights');
  "IW{2,1}(6,:)'" : Constant  Value=[-0.2250425389885272464685073146029026247560977935791015625;-0.74058317615706170666811658520600758492946624755859375;0.348437334605780579810385688688256777822971343994140625;0.340314289282291182470174817353836260735988616943359375;-0.18705217331991896845266865057055838406085968017578125;-1.0233748669572786393899832546594552695751190185546875;0.035666272114076268129334579271016991697251796722412109375;0.5999899674548114791861053163302130997180938720703125;-0.2019365087998765961874170216105994768440723419189453125;0.10737185492537569542204067829516134224832057952880859375;-0.6195191307671592539918492548167705535888671875;0.26669359300381179078698323792195878922939300537109375;-0.766279488225132698886454818421043455600738525390625;0.71480189665993620895534377268631942570209503173828125;0.110964323355941252291501086801872588694095611572265625;1.053472611574683970303567548398859798908233642578125;-0.835807832488919988378484049462713301181793212890625;0.6558085558252042535087866781395860016345977783203125;0.58306932363806740493572533523547463119029998779296875;0.024711823824928959292268615399734699167311191558837890625]
      mask Display: e = 0.06;c1 = [120 150 230]/255;c2 = ([120 150 230]+0)/383;c3 = ([120 150 230]+128)/383;patch([0 1 1 0],[0 0 1 1],c1);patch([0 1 1 1-e 1-e 0+e],[0 0 1 1-e 0+e 0+e],c2);patch([0 0 1 1-e 0+e 0+e],[0 1 1 1-e 1-e 0+e],c3);plot([0 1 1 0 0],[0 0 1 1 0]);disp('weights');
  "IW{2,1}(7,:)'" : Constant  Value=[0.417428204784865031218288322634180076420307159423828125;0.2213133448443756756685019126962288282811641693115234375;0.313006116746481433121829240917577408254146575927734375;-1.101726309136802139931887722923420369625091552734375;0.57129198986179419161857140352367423474788665771484375;-0.0969874848771315745121768259195960126817226409912109375;0.49702484683777548024607995102996937930583953857421875;-0.40139568225476895957370970791089348495006561279296875;-0.63500544228565269921915614759200252592563629150390625;-0.7859100175548967559535640248213894665241241455078125;0.54863782757273593659874677541665732860565185546875;0.040016085437617400499821229686858714558184146881103515625;0.84798063659835143379694955001468770205974578857421875;-0.981060860333789808152005207375623285770416259765625;0.251604628388687245887922472320497035980224609375;0.9900271430624660862207520040101371705532073974609375;-0.3233148996316594914191000498249195516109466552734375;0.13277500892921256792078565922565758228302001953125;-0.2333738669952524491524314953494467772543430328369140625;0.65718581085354033088918868088512681424617767333984375]
      mask Display: e = 0.06;c1 = [120 150 230]/255;c2 = ([120 150 230]+0)/383;c3 = ([120 150 230]+128)/383;patch([0 1 1 0],[0 0 1 1],c1);patch([0 1 1 1-e 1-e 0+e],[0 0 1 1-e 0+e 0+e],c2);patch([0 0 1 1-e 0+e 0+e],[0 1 1 1-e 1-e 0+e],c3);plot([0 1 1 0 0],[0 0 1 1 0]);disp('weights');
  "IW{2,1}(8,:)'" : Constant  Value=[0.7641371394165676900200878662872128188610076904296875;0.719539705132973939072371649672277271747589111328125;1.189609460376156224725718857371248304843902587890625;-0.07412289521530313063379935556440614163875579833984375;-0.048463821471898850534731906236629583872854709625244140625;-0.36743983160692816891668144307914189994335174560546875;-0.24202588027938654047233058008714579045772552490234375;0.293920849686722551741269171543535776436328887939453125;0.1944254026772178345350283734660479240119457244873046875;-0.039234528459279306711326995582567178644239902496337890625;-1.2988220822424449973908622268936596810817718505859375;0.69521090147756747779084207650157622992992401123046875;-1.008936561321522429324204495060257613658905029296875;-0.66503507852874388373010106079163961112499237060546875;-0.218100416769382798864995720578008331358432769775390625;-0.8026700198498522009771249940968118607997894287109375;0.11401092748931064557726955399630242027342319488525390625;0.2498332868426358377433871282846666872501373291015625;-0.293816410342587597259722542730742134153842926025390625;-0.466620929563111574989164864746271632611751556396484375]
      mask Display: e = 0.06;c1 = [120 150 230]/255;c2 = ([120 150 230]+0)/383;c3 = ([120 150 230]+128)/383;patch([0 1 1 0],[0 0 1 1],c1);patch([0 1 1 1-e 1-e 0+e],[0 0 1 1-e 0+e 0+e],c2);patch([0 0 1 1-e 0+e 0+e],[0 1 1 1-e 1-e 0+e],c3);plot([0 1 1 0 0],[0 0 1 1 0]);disp('weights');
  "IW{2,1}(9,:)'" : Constant  Value=[-0.675380560467206070285328678437508642673492431640625;0.414808623195439263309225452758255414664745330810546875;-0.08636082340295990478207244223085581324994564056396484375;-0.052106157557173786443183161054548691026866436004638671875;-0.07956398848703542803217914070046390406787395477294921875;-0.127305413389542321223046883460483513772487640380859375;-0.5601709609834684133744531209231354296207427978515625;0.443339890116264123687273013274534605443477630615234375;0.465868434959147814655722186216735281050205230712890625;-0.271224543033896814403505004520411603152751922607421875;1.1870585121695482744286209708661772310733795166015625;-0.1799409403654457506593900006919284351170063018798828125;0.37670977246739412169773686400731094181537628173828125;0.54335872863801182308662873765570111572742462158203125;0.33654325565796538999308040729374624788761138916015625;0.363035957416277088594114275110769085586071014404296875;-0.53724650019235209441603728919290006160736083984375;-0.387927896247393544371107054757885634899139404296875;-0.025486987172786641775434901546759647317230701446533203125;0.16637141466160676461782941260025836527347564697265625]
      mask Display: e = 0.06;c1 = [120 150 230]/255;c2 = ([120 150 230]+0)/383;c3 = ([120 150 230]+128)/383;patch([0 1 1 0],[0 0 1 1],c1);patch([0 1 1 1-e 1-e 0+e],[0 0 1 1-e 0+e 0+e],c2);patch([0 0 1 1-e 0+e 0+e],[0 1 1 1-e 1-e 0+e],c3);plot([0 1 1 0 0],[0 0 1 1 0]);disp('weights');
  Mux : Mux  Inputs=10
      mask Display: e = 0.06;c1 = [120 150 230]/255;c2 = ([120 150 230]+0)/383;c3 = ([120 150 230]+128)/383;patch([0 1 1 0],[0 0 1 1],c1);patch([0 1 1 1-e 1-e 0+e],[0 0 1 1-e 0+e 0+e],c2);patch([0 0 1 1-e 0+e 0+e],[0 1 1 1-e 1-e 0+e],c3);plot([0 1 1 0 0],[0 0 1 1 0]);disp('Mux');
  dotprod{1..10} (10 alike) : neural/Weight Functions/dotprod
  "lz{2,1}" : Outport
      mask Display: e = 0.06;c1 = [120 230 180]/255;c2 = ([120 230 180]+0)/(256+128);c3 = ([120 230 180]+128)/(256+128);patch([0 1 1 0],[0 0 1 1],c1);patch([0 1 1 1-e 1-e 0+e],[0 0 1 1-e 0+e 0+e],c2);patch([0 0 1 1-e 0+e 0+e],[0 1 1 1-e 1-e 0+e],c3);plot([0 1 1 0 0],[0 0 1 1 0]);
  wires:
  "IW{2,1}(1,:)'"/1 -> dotprod1/1
  "ad{2,1}"/1 -> dotprod1/2, dotprod2/2, dotprod3/2, dotprod4/2, dotprod5/2, dotprod6/2, dotprod7/2, dotprod8/2, dotprod9/2, dotprod10/2
  dotprod1/1 -> Mux/1
  "IW{2,1}(2,:)'"/1 -> dotprod2/1
  dotprod2/1 -> Mux/2
  "IW{2,1}(3,:)'"/1 -> dotprod3/1
  dotprod3/1 -> Mux/3
  "IW{2,1}(4,:)'"/1 -> dotprod4/1
  dotprod4/1 -> Mux/4
  "IW{2,1}(5,:)'"/1 -> dotprod5/1
  dotprod5/1 -> Mux/5
  "IW{2,1}(6,:)'"/1 -> dotprod6/1
  dotprod6/1 -> Mux/6
  "IW{2,1}(7,:)'"/1 -> dotprod7/1
  dotprod7/1 -> Mux/7
  "IW{2,1}(8,:)'"/1 -> dotprod8/1
  dotprod8/1 -> Mux/8
  "IW{2,1}(9,:)'"/1 -> dotprod9/1
  dotprod9/1 -> Mux/9
  "IW{2,1}(10,:)'"/1 -> dotprod10/1
  dotprod10/1 -> Mux/10
  Mux/1 -> "lz{2,1}"/1

== system mrefrobotarm_modified_previous_y_previous_u_previous_ref/no_ss_error/Layer 3/Delays 1 ==
  "p{3}" : Inport  PortDimensions=10
      mask Display: e = 0.06;c1 = [120 230 180]/255;c2 = ([120 230 180]+0)/(256+128);c3 = ([120 230 180]+128)/(256+128);patch([0 1 1 0],[0 0 1 1],c1);patch([0 1 1 1-e 1-e 0+e],[0 0 1 1-e 0+e 0+e],c2);patch([0 0 1 1-e 0+e 0+e],[0 1 1 1-e 1-e 0+e],c3);plot([0 1 1 0 0],[0 0 1 1 0]);
  mux : Mux  Inputs=1
      mask Display: e = 0.06;c1 = [120 150 230]/255;c2 = ([120 150 230]+0)/383;c3 = ([120 150 230]+128)/383;patch([0 1 1 0],[0 0 1 1],c1);patch([0 1 1 1-e 1-e 0+e],[0 0 1 1-e 0+e 0+e],c2);patch([0 0 1 1-e 0+e 0+e],[0 1 1 1-e 1-e 0+e],c3);plot([0 1 1 0 0],[0 0 1 1 0]);disp('Mux')
  "pd{3,2}" : Outport
      mask Display: e = 0.06;c1 = [120 230 180]/255;c2 = ([120 230 180]+0)/(256+128);c3 = ([120 230 180]+128)/(256+128);patch([0 1 1 0],[0 0 1 1],c1);patch([0 1 1 1-e 1-e 0+e],[0 0 1 1-e 0+e 0+e],c2);patch([0 0 1 1-e 0+e 0+e],[0 1 1 1-e 1-e 0+e],c3);plot([0 1 1 0 0],[0 0 1 1 0]);
  wires:
  "p{3}"/1 -> mux/1
  mux/1 -> "pd{3,2}"/1
